simulink model "ES2_simulink"  (R2023b)
settings: Solver=VariableStepAuto  StartTime=0.0  StopTime=30.0  RelTol=1e-3
undefined symbols (not defined in the file): fdesignblkfcn, gcbh
libraries: dspfdesign x4, dspstat3 x4, vrlib x2
settings Model: NumberOfSteps=100  Creator=manu  LastModifiedBy=deluc

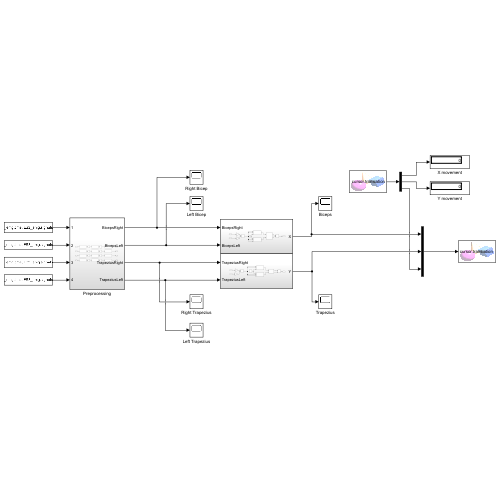
[thumbnail: Simulink's stored preview of the top-level diagram]
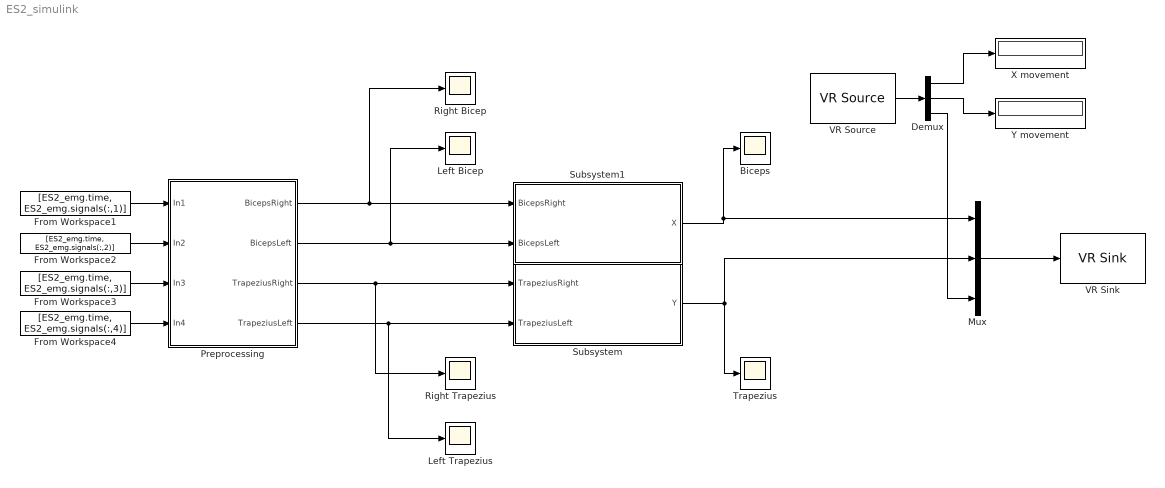
== system ES2_simulink ==
  Biceps : Scope
  Demux : Demux  Outputs=3
  From Workspace1 : FromWorkspace  VariableName=[ES2_emg.time, ES2_emg.signals(:,1)]  OutDataTypeStr=double  SampleTime=0.001
  From Workspace2 : FromWorkspace  VariableName=[ES2_emg.time, ES2_emg.signals(:,2)]  OutDataTypeStr=double  SampleTime=0.001
  From Workspace3 : FromWorkspace  VariableName=[ES2_emg.time, ES2_emg.signals(:,3)]  OutDataTypeStr=double  SampleTime=0.001
  From Workspace4 : FromWorkspace  VariableName=[ES2_emg.time, ES2_emg.signals(:,4)]  OutDataTypeStr=double  SampleTime=0.001
  Left Bicep : Scope
  Left Trapezius : Scope
  Mux : Mux  Inputs=3
  Preprocessing : Subsystem
  Right Bicep : Scope
  Right Trapezius : Scope
  Subsystem : Subsystem
  Subsystem1 : Subsystem
  Trapezius : Scope
  VR Sink : vrlib/VR Sink  InstantiateOnLoad=on  SampleTime=0.1  ViewEnable=on  RemoteChange=off  RemoteView=off  FieldsWritten=cursor.translation.3.1.1.double  WorldFileName=8_palline_color.wrl  AutoView=off  VideoDimensions=[]  AllowVariableSize=off  FigureProperties="{'Position', 'Name', 'Viewpoint', 'CameraBound', 'CameraDirection', 'CameraPosition', 'CameraUpVector', 'ZoomFactor', 'Antialiasing', 'Headlight', 'Lighting', 'NavPanel', 'Sound', 'StatusBar', 'Stereo3D', 'Stereo3DCameraOffset', 'Stereo3DHIT', 'ToolBar', 'Textures', 'Transparency', 'Triad', 'Wireframe', 'NavZones', 'NavMode', 'NavSpeed', 'CaptureFileFormat', 'CaptureFileName', 'Record2DCompressMethod', 'Record2DCompressQuality', 'Record2D', 'Record2DFileName', 'Record2DFPS'; [5.0000000000000000e+00   9.2000000000000000e+01   5.7600000000000000e+02   3.5000000000000000e+02], '', '_untitled_1', 'on', [0.0000000000000000e+00   0.0000000000000000e+00  -1.0000000000000000e+00], [0.0000000000000000e+00   0.0000000000000000e+00   0.0000000000000000e+00], [0.0000000000000000e+00   1.0000000000000000e+00   0.0000000000000000e+00], [1.0000000000000000e+00], 'on', 'on', 'on', 'halfbar', 'on', 'on', 'off', [1.0000000149011612e-01], [0.0000000000000000e+00], 'on', 'on', 'on', 'none', 'off', 'off', 'fly', 'normal', 'tif', '%f_anim_%n.tif', 'auto', [7.5000000000000000e+01], 'off', '%f_anim_%n.avi', 'auto'}"
  VR Source : vrlib/VR Source  InstantiateOnLoad=on  SampleTime=0.1  ViewEnable=on  RemoteChange=off  RemoteView=off  FieldsRead=cursor.translation.1.3.1.double  WorldFileName=8_palline_color.wrl  AutoView=off  VideoDimensions=[]  AllowVariableSize=off
  X movement : Display
  Y movement : Display
  wires:
  From Workspace1/1 -> Preprocessing/1(In1)
  From Workspace2/1 -> Preprocessing/2(In2)
  From Workspace3/1 -> Preprocessing/3(In3)
  From Workspace4/1 -> Preprocessing/4(In4)
  Preprocessing/3(TrapeziusRight) -> Right Trapezius/1, Subsystem/1(TrapeziusRight)
  Preprocessing/4(TrapeziusLeft) -> Left Trapezius/1, Subsystem/2(TrapeziusLeft)
  Preprocessing/1(BicepsRight) -> Right Bicep/1, Subsystem1/1(BicepsRight)
  Preprocessing/2(BicepsLeft) -> Left Bicep/1, Subsystem1/2(BicepsLeft)
  VR Source/1 -> Demux/1
  Demux/3 -> Mux/3
  Demux/1 -> X movement/1
  Demux/2 -> Y movement/1
  Subsystem1/1(X) -> Mux/1, Biceps/1
  Subsystem/1(Y) -> Mux/2, Trapezius/1
  Mux/1 -> VR Sink/1

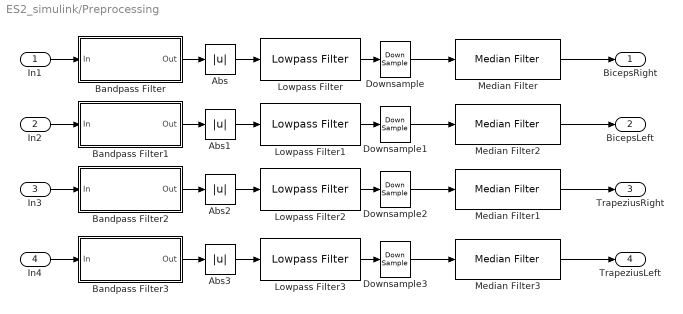
== system ES2_simulink/Preprocessing ==
  In1 : Inport
  In2 : Inport  Port=2
  In3 : Inport  Port=3
  In4 : Inport  Port=4
  Abs{,1..3} (4 alike) : Abs  SaturateOnIntegerOverflow=off
  Bandpass Filter : Subsystem  DialogController=fdesignblkfcn  InitFcn=fdesignblkfcn(gcbh, {'InitFcn'});  mask(Bandpass Filter){}
      mask help: dsp:DSPFilterDesignBlockDialog:BandpassFdesign_MaskDesc
      settings: CopyFcn=fdesignblkfcn(gcbh, {'CopyFcn'});
      mask Help: helpview(mapfilelocation('dsp'), 'dspbandpassfilter');
      mask Display: disp('Bandpass');
  Bandpass Filter1 : Subsystem  DialogController=fdesignblkfcn  InitFcn=fdesignblkfcn(gcbh, {'InitFcn'});  mask(Bandpass Filter){}
      mask help: dsp:DSPFilterDesignBlockDialog:BandpassFdesign_MaskDesc
      settings: CopyFcn=fdesignblkfcn(gcbh, {'CopyFcn'});
      mask Help: helpview(mapfilelocation('dsp'), 'dspbandpassfilter');
      mask Display: disp('Bandpass');
  Bandpass Filter2 : Subsystem  DialogController=fdesignblkfcn  InitFcn=fdesignblkfcn(gcbh, {'InitFcn'});  mask(Bandpass Filter){}
      mask help: dsp:DSPFilterDesignBlockDialog:BandpassFdesign_MaskDesc
      settings: CopyFcn=fdesignblkfcn(gcbh, {'CopyFcn'});
      mask Help: helpview(mapfilelocation('dsp'), 'dspbandpassfilter');
      mask Display: disp('Bandpass');
  Bandpass Filter3 : Subsystem  DialogController=fdesignblkfcn  InitFcn=fdesignblkfcn(gcbh, {'InitFcn'});  mask(Bandpass Filter){}
      mask help: dsp:DSPFilterDesignBlockDialog:BandpassFdesign_MaskDesc
      settings: CopyFcn=fdesignblkfcn(gcbh, {'CopyFcn'});
      mask Help: helpview(mapfilelocation('dsp'), 'dspbandpassfilter');
      mask Display: disp('Bandpass');
  Downsample{,1..3} (4 alike) : DownSample  N=4  RateOptions=Allow multirate processing
  Lowpass Filter{,1..3} (4 alike) : dspfdesign/Lowpass Filter  FilterType=FIR  DesignForMinimumOrder=on  FilterOrder=50  PassbandFrequency=3  StopbandFrequency=6  PassbandRipple=0.1  StopbandAttenuation=80  SampleRateMode=Specify on dialog  SampleRate=1000  SimulateUsing=Interpreted execution  roundingMode=Floor  coeffsDataTypeStr=fixdt(1,16)
  Median Filter : dspstat3/Median Filter  WindowLength=250  SimulateUsing=Interpreted execution
      settings: LibrarySourceBlock=|
      | dspfdesign/Median
      | Filter
  Median Filter1 : dspstat3/Median Filter  WindowLength=300  SimulateUsing=Interpreted execution
      settings: LibrarySourceBlock=|
      | dspfdesign/Median
      | Filter
  Median Filter2 : dspstat3/Median Filter  WindowLength=250  SimulateUsing=Interpreted execution
      settings: LibrarySourceBlock=|
      | dspfdesign/Median
      | Filter
  Median Filter3 : dspstat3/Median Filter  WindowLength=250  SimulateUsing=Interpreted execution
      settings: LibrarySourceBlock=|
      | dspfdesign/Median
      | Filter
  BicepsRight : Outport
  BicepsLeft : Outport  Port=2
  TrapeziusRight : Outport  Port=3
  TrapeziusLeft : Outport  Port=4
  wires:
  Lowpass Filter2/1 -> Downsample2/1
  Bandpass Filter2/1(Out) -> Abs2/1
  Abs1/1 -> Lowpass Filter1/1
  Abs3/1 -> Lowpass Filter3/1
  Abs/1 -> Lowpass Filter/1
  Bandpass Filter3/1(Out) -> Abs3/1
  In4/1 -> Bandpass Filter3/1(In)
  In1/1 -> Bandpass Filter/1(In)
  Bandpass Filter/1(Out) -> Abs/1
  Bandpass Filter1/1(Out) -> Abs1/1
  Abs2/1 -> Lowpass Filter2/1
  Lowpass Filter1/1 -> Downsample1/1
  Lowpass Filter3/1 -> Downsample3/1
  Lowpass Filter/1 -> Downsample/1
  In3/1 -> Bandpass Filter2/1(In)
  In2/1 -> Bandpass Filter1/1(In)
  Downsample/1 -> Median Filter/1
  Downsample1/1 -> Median Filter2/1
  Downsample2/1 -> Median Filter1/1
  Downsample3/1 -> Median Filter3/1
  Median Filter/1 -> BicepsRight/1
  Median Filter2/1 -> BicepsLeft/1
  Median Filter1/1 -> TrapeziusRight/1
  Median Filter3/1 -> TrapeziusLeft/1

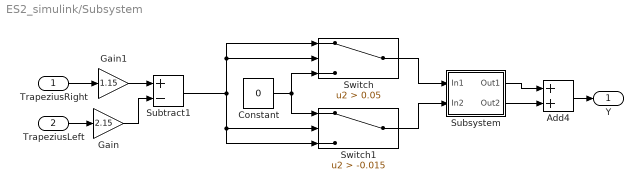
== system ES2_simulink/Subsystem ==
  TrapeziusRight : Inport
  TrapeziusLeft : Inport  Port=2
  Add4 : Sum
  Constant : Constant  Value=0
  Gain : Gain  Gain=2.15
  Gain1 : Gain  Gain=1.15
  Subsystem : Subsystem
  Subtract1 : Sum  Inputs=+-
  Switch : Switch  Criteria=u2 > Threshold  Threshold=0.05  SaturateOnIntegerOverflow=off  InputSameDT=off
  Switch1 : Switch  Criteria=u2 > Threshold  Threshold=-0.015  SaturateOnIntegerOverflow=off  InputSameDT=off
  Y : Outport
  wires:
  TrapeziusLeft/1 -> Gain/1
  Constant/1 -> Switch1/1, Switch/3
  Add4/1 -> Y/1
  Gain/1 -> Subtract1/2
  TrapeziusRight/1 -> Gain1/1
  Subtract1/1 -> Switch1/3, Switch1/2, Switch/1, Switch/2
  Gain1/1 -> Subtract1/1
  Switch/1 -> Subsystem/1(In1)
  Switch1/1 -> Subsystem/2(In2)
  Subsystem/1(Out1) -> Add4/1
  Subsystem/2(Out2) -> Add4/2

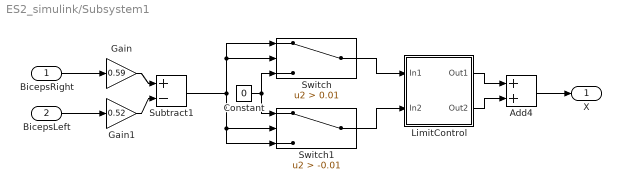
== system ES2_simulink/Subsystem1 ==
  BicepsRight : Inport
  BicepsLeft : Inport  Port=2
  Add4 : Sum
  Constant : Constant  Value=0
  Gain : Gain  Gain=0.59
  Gain1 : Gain  Gain=0.52
  LimitControl : Subsystem
  Subtract1 : Sum  Inputs=+-
  Switch : Switch  Criteria=u2 > Threshold  Threshold=0.01  SaturateOnIntegerOverflow=off  InputSameDT=off
  Switch1 : Switch  Criteria=u2 > Threshold  Threshold=-0.01  SaturateOnIntegerOverflow=off  InputSameDT=off
  X : Outport
  wires:
  BicepsLeft/1 -> Gain1/1
  Subtract1/1 -> Switch1/2, Switch1/3, Switch/1, Switch/2
  BicepsRight/1 -> Gain/1
  Add4/1 -> X/1
  Constant/1 -> Switch1/1, Switch/3
  Gain/1 -> Subtract1/1
  Gain1/1 -> Subtract1/2
  Switch/1 -> LimitControl/1(In1)
  Switch1/1 -> LimitControl/2(In2)
  LimitControl/1(Out1) -> Add4/1
  LimitControl/2(Out2) -> Add4/2

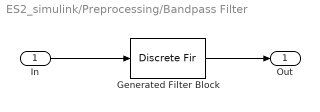
== system ES2_simulink/Preprocessing/Bandpass Filter ==
  In : Inport
  Generated Filter Block : DiscreteFir  Tag=BlockMethodSubSystem  Coefficients=[8.09984662039171649e-19 6.39138873735446358e-05 -0.000529985360713195928 0.000163049509978641067 -0.0010687365606513342 0.00013845410762377186 -0.0015074021939330644 -0.000146171169312382047 -0.00164491285071874773 -0.000803831165663842638 -0.0012700293910364235 -0.00179475969145176514 -0.00031320271539095237 -0.0028004705363883697 0.00102378750565708691 -0.00320898606072516409 0.00226847122552957916 -0.00229118992766688288 0.0028627312851967927 0.000444283590646493373 0.00248061645378651156 0.00484772649949967351 0.00132315559732985649 0.00988516690279818248 0.000195375038696813568 0.0137475146561206601 0.000235578061564315101 0.0143783789118080065 0.00232373851233996223 0.0102932854869860861 0.00637980828249819915 0.00138721018355516027 0.0108821641584976002 -0.0106388069047137195 0.0129164407258159069 -0.0225052497171089674 0.00888838159476280747 -0.030269754297304826 -0.00424164083303872706 -0.0306714306083059572 -0.0276065409272709984 -0.0224239239611803629 -0.0594922495550082794 -0.00693651358874993514 -0.0952531612511481052 0.0118816213758879945 -0.128243809353299099 0.0287429432612044122 -0.151547652016043616 0.0386729267839347329 0.839787881504185374 0.0386729267839347329 -0.151547652016043616 0.0287429432612044122 -0.128243809353299099 0.0118816213758879945 -0.0952531612511481052 -0.00693651358874993514 -0.0594922495550082794 -0.0224239239611803629 -0.0276065409272709984 -0.0306714306083059572 -0.00424164083303872706 -0.030269754297304826 0.00888838159476280747 -0.0225052497171089674 0.0129164407258159069 -0.0106388069047137195 0.0108821641584976002 0.00138721018355516027 0.00637980828249819915 0.0102932854869860861 0.00232373851233996223 0.0143783789118080065 0.000235578061564315101 0.0137475146561206601 0.000195375038696813568 0.00988516690279818248 0.00132315559732985649 0.00484772649949967351 0.00248061645378651156 0.000444283590646493373 0.0028627312851967927 -0.00229118992766688288 0.00226847122552957916 -0.00320898606072516409 0.00102378750565708691 -0.0028004705363883697 -0.00031320271539095237 -0.00179475969145176514 -0.0012700293910364235 -0.000803831165663842638 -0.00164491285071874773 -0.000146171169312382047 -0.0015074021939330644 0.00013845410762377186 -0.0010687365606513342 0.000163049509978641067 -0.000529985360713195928 6.39138873735446358e-05 8.09984662039171649e-19]  InputProcessing=Columns as channels (frame based)
  Out : Outport  VectorParamsAs1DForOutWhenUnconnected=off
  wires:
  In/1 -> Generated Filter Block/1
  Generated Filter Block/1 -> Out/1

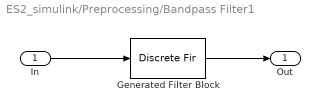
== system ES2_simulink/Preprocessing/Bandpass Filter1 ==
  In : Inport
  Generated Filter Block : DiscreteFir  Tag=BlockMethodSubSystem  Coefficients=[8.09984662039171649e-19 6.39138873735446358e-05 -0.000529985360713195928 0.000163049509978641067 -0.0010687365606513342 0.00013845410762377186 -0.0015074021939330644 -0.000146171169312382047 -0.00164491285071874773 -0.000803831165663842638 -0.0012700293910364235 -0.00179475969145176514 -0.00031320271539095237 -0.0028004705363883697 0.00102378750565708691 -0.00320898606072516409 0.00226847122552957916 -0.00229118992766688288 0.0028627312851967927 0.000444283590646493373 0.00248061645378651156 0.00484772649949967351 0.00132315559732985649 0.00988516690279818248 0.000195375038696813568 0.0137475146561206601 0.000235578061564315101 0.0143783789118080065 0.00232373851233996223 0.0102932854869860861 0.00637980828249819915 0.00138721018355516027 0.0108821641584976002 -0.0106388069047137195 0.0129164407258159069 -0.0225052497171089674 0.00888838159476280747 -0.030269754297304826 -0.00424164083303872706 -0.0306714306083059572 -0.0276065409272709984 -0.0224239239611803629 -0.0594922495550082794 -0.00693651358874993514 -0.0952531612511481052 0.0118816213758879945 -0.128243809353299099 0.0287429432612044122 -0.151547652016043616 0.0386729267839347329 0.839787881504185374 0.0386729267839347329 -0.151547652016043616 0.0287429432612044122 -0.128243809353299099 0.0118816213758879945 -0.0952531612511481052 -0.00693651358874993514 -0.0594922495550082794 -0.0224239239611803629 -0.0276065409272709984 -0.0306714306083059572 -0.00424164083303872706 -0.030269754297304826 0.00888838159476280747 -0.0225052497171089674 0.0129164407258159069 -0.0106388069047137195 0.0108821641584976002 0.00138721018355516027 0.00637980828249819915 0.0102932854869860861 0.00232373851233996223 0.0143783789118080065 0.000235578061564315101 0.0137475146561206601 0.000195375038696813568 0.00988516690279818248 0.00132315559732985649 0.00484772649949967351 0.00248061645378651156 0.000444283590646493373 0.0028627312851967927 -0.00229118992766688288 0.00226847122552957916 -0.00320898606072516409 0.00102378750565708691 -0.0028004705363883697 -0.00031320271539095237 -0.00179475969145176514 -0.0012700293910364235 -0.000803831165663842638 -0.00164491285071874773 -0.000146171169312382047 -0.0015074021939330644 0.00013845410762377186 -0.0010687365606513342 0.000163049509978641067 -0.000529985360713195928 6.39138873735446358e-05 8.09984662039171649e-19]  InputProcessing=Columns as channels (frame based)
  Out : Outport  VectorParamsAs1DForOutWhenUnconnected=off
  wires:
  In/1 -> Generated Filter Block/1
  Generated Filter Block/1 -> Out/1

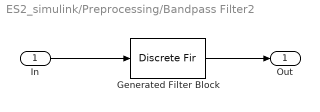
== system ES2_simulink/Preprocessing/Bandpass Filter2 ==
  In : Inport
  Generated Filter Block : DiscreteFir  Tag=BlockMethodSubSystem  Coefficients=[8.09984662039171649e-19 6.39138873735446358e-05 -0.000529985360713195928 0.000163049509978641067 -0.0010687365606513342 0.00013845410762377186 -0.0015074021939330644 -0.000146171169312382047 -0.00164491285071874773 -0.000803831165663842638 -0.0012700293910364235 -0.00179475969145176514 -0.00031320271539095237 -0.0028004705363883697 0.00102378750565708691 -0.00320898606072516409 0.00226847122552957916 -0.00229118992766688288 0.0028627312851967927 0.000444283590646493373 0.00248061645378651156 0.00484772649949967351 0.00132315559732985649 0.00988516690279818248 0.000195375038696813568 0.0137475146561206601 0.000235578061564315101 0.0143783789118080065 0.00232373851233996223 0.0102932854869860861 0.00637980828249819915 0.00138721018355516027 0.0108821641584976002 -0.0106388069047137195 0.0129164407258159069 -0.0225052497171089674 0.00888838159476280747 -0.030269754297304826 -0.00424164083303872706 -0.0306714306083059572 -0.0276065409272709984 -0.0224239239611803629 -0.0594922495550082794 -0.00693651358874993514 -0.0952531612511481052 0.0118816213758879945 -0.128243809353299099 0.0287429432612044122 -0.151547652016043616 0.0386729267839347329 0.839787881504185374 0.0386729267839347329 -0.151547652016043616 0.0287429432612044122 -0.128243809353299099 0.0118816213758879945 -0.0952531612511481052 -0.00693651358874993514 -0.0594922495550082794 -0.0224239239611803629 -0.0276065409272709984 -0.0306714306083059572 -0.00424164083303872706 -0.030269754297304826 0.00888838159476280747 -0.0225052497171089674 0.0129164407258159069 -0.0106388069047137195 0.0108821641584976002 0.00138721018355516027 0.00637980828249819915 0.0102932854869860861 0.00232373851233996223 0.0143783789118080065 0.000235578061564315101 0.0137475146561206601 0.000195375038696813568 0.00988516690279818248 0.00132315559732985649 0.00484772649949967351 0.00248061645378651156 0.000444283590646493373 0.0028627312851967927 -0.00229118992766688288 0.00226847122552957916 -0.00320898606072516409 0.00102378750565708691 -0.0028004705363883697 -0.00031320271539095237 -0.00179475969145176514 -0.0012700293910364235 -0.000803831165663842638 -0.00164491285071874773 -0.000146171169312382047 -0.0015074021939330644 0.00013845410762377186 -0.0010687365606513342 0.000163049509978641067 -0.000529985360713195928 6.39138873735446358e-05 8.09984662039171649e-19]  InputProcessing=Columns as channels (frame based)
  Out : Outport  VectorParamsAs1DForOutWhenUnconnected=off
  wires:
  In/1 -> Generated Filter Block/1
  Generated Filter Block/1 -> Out/1

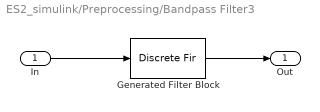
== system ES2_simulink/Preprocessing/Bandpass Filter3 ==
  In : Inport
  Generated Filter Block : DiscreteFir  Tag=BlockMethodSubSystem  Coefficients=[8.09984662039171649e-19 6.39138873735446358e-05 -0.000529985360713195928 0.000163049509978641067 -0.0010687365606513342 0.00013845410762377186 -0.0015074021939330644 -0.000146171169312382047 -0.00164491285071874773 -0.000803831165663842638 -0.0012700293910364235 -0.00179475969145176514 -0.00031320271539095237 -0.0028004705363883697 0.00102378750565708691 -0.00320898606072516409 0.00226847122552957916 -0.00229118992766688288 0.0028627312851967927 0.000444283590646493373 0.00248061645378651156 0.00484772649949967351 0.00132315559732985649 0.00988516690279818248 0.000195375038696813568 0.0137475146561206601 0.000235578061564315101 0.0143783789118080065 0.00232373851233996223 0.0102932854869860861 0.00637980828249819915 0.00138721018355516027 0.0108821641584976002 -0.0106388069047137195 0.0129164407258159069 -0.0225052497171089674 0.00888838159476280747 -0.030269754297304826 -0.00424164083303872706 -0.0306714306083059572 -0.0276065409272709984 -0.0224239239611803629 -0.0594922495550082794 -0.00693651358874993514 -0.0952531612511481052 0.0118816213758879945 -0.128243809353299099 0.0287429432612044122 -0.151547652016043616 0.0386729267839347329 0.839787881504185374 0.0386729267839347329 -0.151547652016043616 0.0287429432612044122 -0.128243809353299099 0.0118816213758879945 -0.0952531612511481052 -0.00693651358874993514 -0.0594922495550082794 -0.0224239239611803629 -0.0276065409272709984 -0.0306714306083059572 -0.00424164083303872706 -0.030269754297304826 0.00888838159476280747 -0.0225052497171089674 0.0129164407258159069 -0.0106388069047137195 0.0108821641584976002 0.00138721018355516027 0.00637980828249819915 0.0102932854869860861 0.00232373851233996223 0.0143783789118080065 0.000235578061564315101 0.0137475146561206601 0.000195375038696813568 0.00988516690279818248 0.00132315559732985649 0.00484772649949967351 0.00248061645378651156 0.000444283590646493373 0.0028627312851967927 -0.00229118992766688288 0.00226847122552957916 -0.00320898606072516409 0.00102378750565708691 -0.0028004705363883697 -0.00031320271539095237 -0.00179475969145176514 -0.0012700293910364235 -0.000803831165663842638 -0.00164491285071874773 -0.000146171169312382047 -0.0015074021939330644 0.00013845410762377186 -0.0010687365606513342 0.000163049509978641067 -0.000529985360713195928 6.39138873735446358e-05 8.09984662039171649e-19]  InputProcessing=Columns as channels (frame based)
  Out : Outport  VectorParamsAs1DForOutWhenUnconnected=off
  wires:
  In/1 -> Generated Filter Block/1
  Generated Filter Block/1 -> Out/1

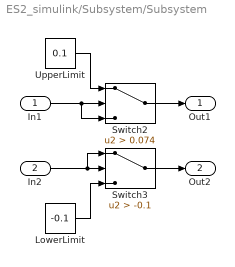
== system ES2_simulink/Subsystem/Subsystem ==
  In1 : Inport
  In2 : Inport  Port=2
  LowerLimit : Constant  Value=-0.1
  Switch2 : Switch  Criteria=u2 > Threshold  Threshold=0.074  SaturateOnIntegerOverflow=off  InputSameDT=off
  Switch3 : Switch  Criteria=u2 > Threshold  Threshold=-0.1  SaturateOnIntegerOverflow=off  InputSameDT=off
  UpperLimit : Constant  Value=0.1
  Out1 : Outport
  Out2 : Outport  Port=2
  wires:
  In2/1 -> Switch3/1, Switch3/2
  In1/1 -> Switch2/3, Switch2/2
  LowerLimit/1 -> Switch3/3
  Switch2/1 -> Out1/1
  UpperLimit/1 -> Switch2/1
  Switch3/1 -> Out2/1

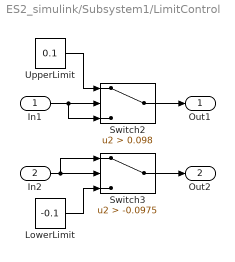
== system ES2_simulink/Subsystem1/LimitControl ==
  In1 : Inport
  In2 : Inport  Port=2
  LowerLimit : Constant  Value=-0.1
  Switch2 : Switch  Criteria=u2 > Threshold  Threshold=0.098  SaturateOnIntegerOverflow=off  InputSameDT=off
  Switch3 : Switch  Criteria=u2 > Threshold  Threshold=-0.0975  SaturateOnIntegerOverflow=off  InputSameDT=off
  UpperLimit : Constant  Value=0.1
  Out1 : Outport
  Out2 : Outport  Port=2
  wires:
  In2/1 -> Switch3/1, Switch3/2
  UpperLimit/1 -> Switch2/1
  LowerLimit/1 -> Switch3/3
  In1/1 -> Switch2/3, Switch2/2
  Switch3/1 -> Out2/1
  Switch2/1 -> Out1/1
